simulink model "atomicVsVirtual"  (R2018a)
settings: Solver=FixedStepDiscrete  StartTime=0.0  StopTime=10.0  RelTol=1e-3  EnableMultiTasking=on
settings Model: Creator=jrivitus  LastModifiedBy=bneiswan
settings DataIOCC: LimitDataPoints=on  SaveFormat=Array
settings OptimizationCC: ExpressionDepthLimit=2147483647  LifeSpan=inf
settings DebuggingCC: UnderspecifiedInitializationDetection=Classic  MergeDetectMultiDrivingBlocksExec=none  ParameterPrecisionLossMsg=none  FcnCallInpInsideContextMsg=warning  AllowSymbolicDim=off  StateNameClashWarn=warning  SFUnexpectedBacktrackingDiag=warning  SFNoUnconditionalDefaultTransitionDiag=warning  SFExecutionAtInitializationDiag=none
settings HardwareCC: ProdBitPerPointer=32  ProdBitPerSizeT=32  ProdBitPerPtrDiffT=32  ProdLargestAtomicFloat=None  ProdIntDivRoundTo=Undefined  ProdEndianess=Unspecified  ProdWordSize=32  ProdHWDeviceType=32-bit Generic
settings ModelReferenceCC: PropagateSignalLabelsOutOfModel=off
settings CodeAppCC: StateflowObjectComments=on
settings GRTTargetCC: TargetLangStandard=C89/C90 (ANSI)  GeneratePreprocessorConditionals=Disable all  CombineOutputUpdateFcns=off  GRTInterface=on
settings ConfigComp: CovMetricSettings=dw  CovHtmlReporting=on  CovSaveCumulativeToWorkspaceVar=on  CovSaveSingleToWorkspaceVar=on  CovExternalEMLEnable=off  CovSFcnEnable=off

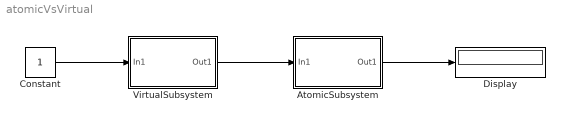
== system atomicVsVirtual ==
  AtomicSubsystem : Subsystem  TreatAsAtomicUnit=on
  Constant : Constant  SampleTime=0.1
  Display : Display
  VirtualSubsystem : Subsystem
  wires:
  Constant/1 -> VirtualSubsystem/1(In1)
  VirtualSubsystem/1(Out1) -> AtomicSubsystem/1(In1)
  AtomicSubsystem/1(Out1) -> Display/1

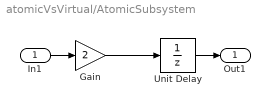
== system atomicVsVirtual/AtomicSubsystem ==
  In1 : Inport
  Gain : Gain  Gain=2
  Unit Delay : UnitDelay  SampleTime=-1
  Out1 : Outport
  wires:
  Unit Delay/1 -> Out1/1
  In1/1 -> Gain/1
  Gain/1 -> Unit Delay/1

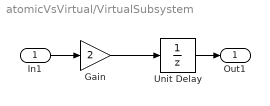
== system atomicVsVirtual/VirtualSubsystem ==
  In1 : Inport
  Gain : Gain  Gain=2
  Unit Delay : UnitDelay  SampleTime=-1
  Out1 : Outport
  wires:
  Gain/1 -> Unit Delay/1
  In1/1 -> Gain/1
  Unit Delay/1 -> Out1/1
